simulink model "delay_test"  (R2019a)
settings: Solver=VariableStepAuto  StartTime=0.0  StopTime=512  RelTol=1e-3
libraries: xbsIndex_r4 x3559
(part 1 of 23)
settings Model: Creator=jackh  LastModifiedBy=jackh

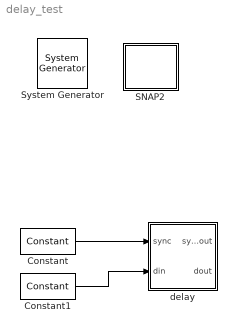
== system delay_test ==
  " System Generator" : xbsIndex_r4/ System Generator  Tag=genX  xilinxfamily=kintexu  part=xcku115  speed=-2-e  package=flvf1924  synthesis_tool=XST  clock_wrapper=Clock Enables  directory=/home/jackh/src/caltech-lwa/snap2_f_200msps_64i_4096c/sysgen  proj_type=Vivado  Synth_file=Vivado Synthesis Defaults  Impl_file=Vivado Implementation Defaults  testbench=off  simulink_period=1  sysclk_period=5  dcm_input_clock_period=10  incr_netlist=off  trim_vbits=Everywhere in SubSystem  dbl_ovrd=According to Block Masks  core_generation=According to Block Masks  run_coregen=off  deprecated_control=off  eval_field=0  block_type=sysgen
  Constant : xbsIndex_r4/Constant  const=0  gui_display_data_type=Boolean  arith_type=Boolean  n_bits=16  bin_pt=14  preci_type=Single  exp_width=8  frac_width=24  explicit_period=on  period=1  equ=P=C  opselect=C  inp2=PCIN>>17  opr=+  inp1=P  carry=CIN  dbl_ovrd=off  block_type=constant
  Constant1 : xbsIndex_r4/Constant  const=0  gui_display_data_type=Fixed-point  arith_type=Unsigned  n_bits=10*64  bin_pt=14  preci_type=Single  exp_width=8  frac_width=24  explicit_period=on  period=1  equ=P=C  opselect=C  inp2=PCIN>>17  opr=+  inp1=P  carry=CIN  dbl_ovrd=off  block_type=constant
  SNAP2 : Subsystem  Tag=xps:xsg  mask(xsg core config){hw_sys=SNAP2_v2:xcku115, clk_src=adc1_clk, clk_rate=200, use_microblaze=on, sample_period=1, synthesis_tool=XST}
      mask prompts: hw_sys "Hardware Platform"; clk_src "User IP Clock source"; clk_rate "User IP Clock Rate (MHz)"; use_microblaze "Use Microblaze controller?"; sample_period "Sample Period"; synthesis_tool "Synthesis Tool:"
      mask help:
      | The XSG Core Config block is used to configure the System Generator design
      | for the casper_xps toolflow. Settings here are used to configure the
      | Xilinx System Generator block parameters automatically, and control toolflow
      | script  execution. It needs to be at the top level of all designs being compiled
      | with the casper_xps toolflow.
      mask init:
      | xps_xsg_snap2_conf_mask;
      mask Help: eval('xlWeb([getenv(''MLIB_ROOT''), ''\doc\html\sys_xsg_core_config\sys_xsg_core_config.html''])')
      mask TypeOptions hw_sys: SNAP2_v1:xcku115 | SNAP2_v2:xcku115
      mask TypeOptions clk_src: sys_clk | clk_250MHz | adc0_clk | adc1_clk
      mask TypeOptions synthesis_tool: Leonardo Spectrum | Synplify | Synplify Pro | XST
      mask Display: fprintf(['SNAP2']);
  delay : Subsystem  mask{max_delay_bits=13}
      mask prompts: max_delay_bits "Manimum delay (2^?) samples"
  wires:
  Constant/1 -> delay/1(sync)
  Constant1/1 -> delay/2(din)

== system delay_test/SNAP2 ==

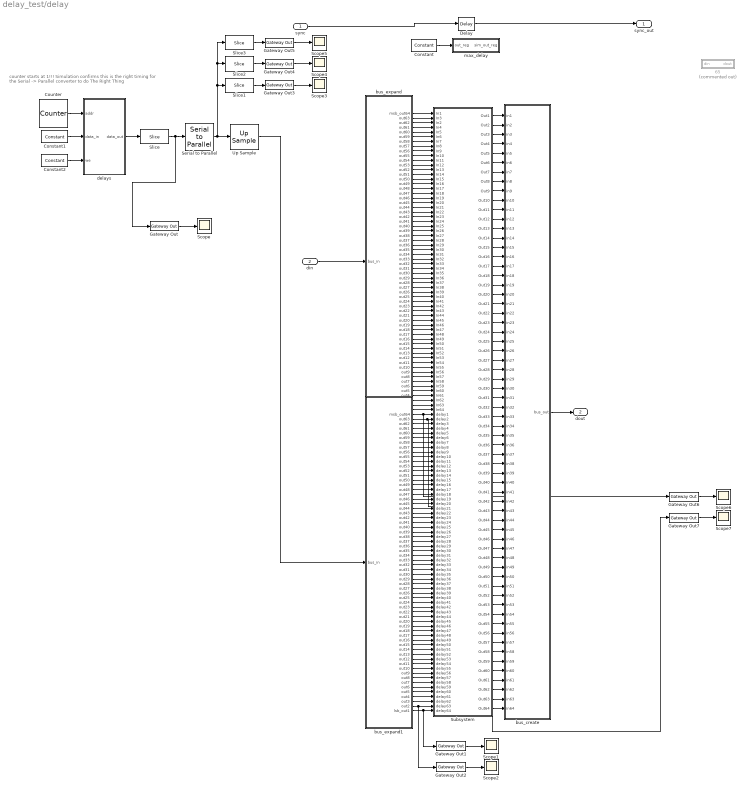
== system delay_test/delay ==
  note: counter starts at 1!!!
      | Simulation confirms this is the right
      | timing for the Serial -> Parallel converter to do The Right Thing
  sync : Inport
  din : Inport  Port=2
  65 : Subsystem  Commented=on
  Constant : xbsIndex_r4/Constant  const=2^max_delay_bits  gui_display_data_type=Fixed-point  arith_type=Unsigned  n_bits=32  bin_pt=0  preci_type=Single  exp_width=8  frac_width=24  explicit_period=on  period=1  equ=P=C  opselect=C  inp2=PCIN>>17  opr=+  inp1=P  carry=CIN  dbl_ovrd=off  block_type=constant
  Constant1 : xbsIndex_r4/Constant  const=0  gui_display_data_type=Fixed-point  arith_type=Unsigned  n_bits=32  bin_pt=0  preci_type=Single  exp_width=8  frac_width=24  explicit_period=on  period=1  equ=P=C  opselect=C  inp2=PCIN>>17  opr=+  inp1=P  carry=CIN  dbl_ovrd=off  block_type=constant
  Constant2 : xbsIndex_r4/Constant  const=0  gui_display_data_type=Boolean  arith_type=Boolean  n_bits=32  bin_pt=0  preci_type=Single  exp_width=8  frac_width=24  explicit_period=on  period=1  equ=P=C  opselect=C  inp2=PCIN>>17  opr=+  inp1=P  carry=CIN  dbl_ovrd=off  block_type=constant
  Counter : xbsIndex_r4/Counter  cnt_type=Free Running  cnt_to=Inf  operation=Up  start_count=1  cnt_by_val=1  arith_type=Unsigned  n_bits=6  bin_pt=0  load_pin=off  rst=off  en=off  explicit_period=on  period=1  use_behavioral_HDL=off  implementation=Fabric  dbl_ovrd=off  block_type=counter
  Delay : xbsIndex_r4/Delay  rst=off  infoeditControl=Selection of Reset will increase slice count due to use of real FFs and instead of SRLs  en=off  latency=7  reg_retiming=on  dbl_ovrd=off  block_type=delay
  Gateway Out{,1..7} (8 alike) : xbsIndex_r4/Gateway Out  inherit_from_input=off  hdl_port=off  rows=1  columns=1  UseAsDAC=off  DACChannel='1'  interface=None  automatic_assignment=on  address_offset=hex2dec('00')  intf_name=''  intf_description=''  timing_constraint=None  locs_specified=off  LOCs={}  io_standard={}  block_type=gatewayout
  Scope{,1..7} (8 alike) : Scope
  Serial to Parallel : xbsIndex_r4/Serial to Parallel  input_order=Most Significant Word First  arith_type=Unsigned  output_bits=13*64  bin_pt=0  rst=off  en=off  latency=1  dbl_ovrd=off  block_type=s2p
      settings: infoedit=Groups of samples presented serially at the input become single samples presented at the output.
  Slice : xbsIndex_r4/Slice  nbits=13  boolean_output=off  mode=Lower Bit Location + Width  bit1=0  base1=MSB of Input  bit0=0  base0=LSB of Input  dbl_ovrd=off  block_type=slice
  Slice1 : xbsIndex_r4/Slice  nbits=13  boolean_output=off  mode=Lower Bit Location + Width  bit1=0  base1=MSB of Input  bit0=0  base0=LSB of Input  dbl_ovrd=off  block_type=slice
  Slice2 : xbsIndex_r4/Slice  nbits=13  boolean_output=off  mode=Lower Bit Location + Width  bit1=0  base1=MSB of Input  bit0=13  base0=LSB of Input  dbl_ovrd=off  block_type=slice
  Slice3 : xbsIndex_r4/Slice  nbits=13  boolean_output=off  mode=Lower Bit Location + Width  bit1=0  base1=MSB of Input  bit0=13*2  base0=LSB of Input  dbl_ovrd=off  block_type=slice
  Subsystem : Subsystem
  Up Sample : xbsIndex_r4/Up Sample  sample_ratio=64  copy_samples=on  en=off  latency=1  dbl_ovrd=off  block_type=usamp
  bus_create : Subsystem  AncestorBlock=casper_library_flow_control/bus_create  mask(bus_create){inputNum=64}
      mask prompts: inputNum "Number of inputs:"
      mask init:
      | bus_create_init(gcb,...
      |     'inputNum', inputNum);
  bus_expand : Subsystem  AncestorBlock=casper_library_flow_control/bus_expand  mask(bus_expand){mode=divisions of equal size, outputNum=8*8, outputWidth=10, outputBinaryPt=0, outputArithmeticType=0, show_format=off, outputToWorkspace=off, variablePrefix=out, outputToModelAsWell=on}
      mask prompts: outputNum "Number of outputs:"; outputWidth "Output width:"; outputBinaryPt "Output binary point position:"; outputArithmeticType "Output arithmetic type (ufix=0, fix=1, bool=2):"; show_format "Print format string?"; outputToWorkspace "Output to workspace?"; variablePrefix "Variable name prefix:"; outputToModelAsWell "Output to model as well?"
      mask help:
      | Expands a 'bus' made using a bus_create or Xilinx
      | concat block.
      | The input will be divided into the specified number
      | of outputs with the specified arithmetic types.
      | Divisions are made from most significant bit.
      mask init:
      | bus_expand_init(gcb,...
      |     'mode', mode, ...
      |     'outputNum', outputNum, ...
      |     'outputWidth', outputWidth, ...
      |     'outputBinaryPt', outputBinaryPt, ...
      |     'outputArithmeticType', outputArithmeticType, ...
      |     'show_format', show_format, ...
      |     'outputToWorkspace', outputToWorkspace, ...
      |     'variablePrefix', variablePrefix, ...
      |     'outputToModelAsWell', outputToModelAsWell);
      settings: AttributesFormatString=64 outputs
      mask TypeOptions mode: divisions of equal size | divisions of arbitrary size
      mask Callback mode: bus_expand_callback();
      mask Callback outputWidth: bus_expand_callback();
      mask Callback outputToWorkspace: bus_expand_callback();
  bus_expand1 : Subsystem  AncestorBlock=casper_library_flow_control/bus_expand  mask(bus_expand){mode=divisions of equal size, outputNum=8*8, outputWidth=13, outputBinaryPt=0, outputArithmeticType=0, show_format=off, outputToWorkspace=off, variablePrefix=out, outputToModelAsWell=on}
      mask prompts: outputNum "Number of outputs:"; outputWidth "Output width:"; outputBinaryPt "Output binary point position:"; outputArithmeticType "Output arithmetic type (ufix=0, fix=1, bool=2):"; show_format "Print format string?"; outputToWorkspace "Output to workspace?"; variablePrefix "Variable name prefix:"; outputToModelAsWell "Output to model as well?"
      mask help:
      | Expands a 'bus' made using a bus_create or Xilinx
      | concat block.
      | The input will be divided into the specified number
      | of outputs with the specified arithmetic types.
      | Divisions are made from most significant bit.
      mask init: same as delay_test/delay/bus_expand
      settings: AttributesFormatString=64 outputs
      mask TypeOptions mode: divisions of equal size | divisions of arbitrary size
      mask Callback mode: bus_expand_callback();
      mask Callback outputWidth: bus_expand_callback();
      mask Callback outputToWorkspace: bus_expand_callback();
  delays : Subsystem  Tag=xps:bram  AncestorBlock=xps_library/Memory/shared_bram  mask{sample_rate=1, init_vals=[0:2^6-1], data_bin_pt=0, optimization=Minimum_Area, reg_core_output=off, reg_prim_output=off, data_width=32, addr_width=6, arith_type=Unsigned, desc_str="", type_desc=""}
      mask prompts: sample_rate "Sample rate"; init_vals "Initial values (simulation only)"; data_bin_pt "Data Binary Point"; reg_core_output "Register Core Output"; reg_prim_output "Register Primitive Output"; data_width "Data Width"; addr_width "Address width"; arith_type "Output Data Type"; desc_str "Description"; type_desc "Word Type Description"
      mask init:
      | shared_bram_mask;
      mask TypeOptions optimization: Minimum_Area | Low_Power
      mask TypeOptions data_width: 8 | 16 | 32 | 64 | 128
      mask TypeOptions arith_type: Unsigned | Signed  (2's comp)
      mask DialogControl Container4 Prompt: Configuration
      mask DialogControl Container10 Prompt: Documentation
  max_delay : Subsystem  Tag=xps:sw_reg  AncestorBlock=xps_library/Memory/software_register  mask(swreg){io_dir=To Processor, io_delay=0, init_val=0, sample_period=1, names=reg, bitwidths=32, bin_pts=0, arith_types=0, sim_port=on, show_format=off, desc_str=|}
      mask desc_str=|
      | Interpretted as a unint32 value, contains the maximum
      | allowed delay, in ADC samples, which may be applied
      | to a data stream.
      mask prompts: io_dir "I/O direction"; io_delay "I/O delay"; init_val "Initial Value"; sample_period "Sample period"; names "Bitfield names [msb...lsb]"; bitwidths "Bitfield widths"; bin_pts "Bitfield binary pts"; arith_types "Bitfield types, ufix=0, fix=1, bool=2"; sim_port "Provide sim input/output?"; show_format "Print format string?"; desc_str "Description"
      mask help: A 32-bit software-accessible register. Can be divided into bitfields of varying widths and types using the fields in the block mask.
      mask init:
      | swreg_init(gcb)
      settings: AttributesFormatString=1output
      mask TypeOptions io_dir: To Processor | From Processor
      mask Callback io_dir:
      | mask_enables = get_param(gcb, 'MaskEnables');
      | mask_names = get_param(gcb, 'MaskNames');
      | if strcmp(get_param(gcb, 'io_dir'), 'To Processor'),
      |     mask_enables{ismember(mask_names, 'sample_period')} = 'off';
      | else
      |     mask_enables{ismember(mask_names, 'sample_period')} = 'on';
      | end
      | set_param(gcb, 'MaskEnables', mask_enables);
      mask DialogControl ParameterTabVar0 Prompt: Setup
  sync_out : Outport
  dout : Outport  Port=2
  wires:
  sync/1 -> Delay/1
  din/1 -> bus_expand/1(bus_in)
  bus_create/1(bus_out) -> dout/1
  Constant/1 -> max_delay/1(out_reg)
  Delay/1 -> sync_out/1
  Counter/1 -> delays/1(addr)
  Constant1/1 -> delays/2(data_in)
  Constant2/1 -> delays/3(we)
  delays/1(data_out) -> Slice/1
  Serial to Parallel/1 -> Up Sample/1, Slice3/1, Slice2/1, Slice1/1
  Slice/1 -> Gateway Out/1, Serial to Parallel/1
  Up Sample/1 -> bus_expand1/1(bus_in)
  Subsystem/1(Out1) -> bus_create/1(in1)
  Subsystem/2(Out2) -> bus_create/2(in2)
  Subsystem/3(Out3) -> bus_create/3(in3)
  Subsystem/4(Out4) -> bus_create/4(in4)
  Subsystem/5(Out5) -> bus_create/5(in5)
  Subsystem/6(Out6) -> bus_create/6(in6)
  Subsystem/7(Out7) -> bus_create/7(in7)
  Subsystem/8(Out8) -> bus_create/8(in8)
  Subsystem/9(Out9) -> bus_create/9(in9)
  Subsystem/10(Out10) -> bus_create/10(in10)
  Subsystem/11(Out11) -> bus_create/11(in11)
  Subsystem/12(Out12) -> bus_create/12(in12)
  Subsystem/13(Out13) -> bus_create/13(in13)
  Subsystem/14(Out14) -> bus_create/14(in14)
  Subsystem/15(Out15) -> bus_create/15(in15)
  Subsystem/16(Out16) -> bus_create/16(in16)
  Subsystem/17(Out17) -> bus_create/17(in17)
  Subsystem/18(Out18) -> bus_create/18(in18)
  Subsystem/19(Out19) -> bus_create/19(in19)
  Subsystem/20(Out20) -> bus_create/20(in20)
  Subsystem/21(Out21) -> bus_create/21(in21)
  Subsystem/22(Out22) -> bus_create/22(in22)
  Subsystem/23(Out23) -> bus_create/23(in23)
  Subsystem/24(Out24) -> bus_create/24(in24)
  Subsystem/25(Out25) -> bus_create/25(in25)
  Subsystem/26(Out26) -> bus_create/26(in26)
  Subsystem/27(Out27) -> bus_create/27(in27)
  Subsystem/28(Out28) -> bus_create/28(in28)
  Subsystem/29(Out29) -> bus_create/29(in29)
  Subsystem/30(Out30) -> bus_create/30(in30)
  Subsystem/31(Out31) -> bus_create/31(in31)
  Subsystem/32(Out32) -> bus_create/32(in32)
  Subsystem/33(Out33) -> bus_create/33(in33)
  Subsystem/34(Out34) -> bus_create/34(in34)
  Subsystem/35(Out35) -> bus_create/35(in35)
  Subsystem/36(Out36) -> bus_create/36(in36)
  Subsystem/37(Out37) -> bus_create/37(in37)
  Subsystem/38(Out38) -> bus_create/38(in38)
  Subsystem/39(Out39) -> bus_create/39(in39)
  Subsystem/40(Out40) -> bus_create/40(in40)
  Subsystem/41(Out41) -> bus_create/41(in41)
  Subsystem/42(Out42) -> bus_create/42(in42)
  Subsystem/43(Out43) -> bus_create/43(in43)
  Subsystem/44(Out44) -> bus_create/44(in44)
  Subsystem/45(Out45) -> bus_create/45(in45)
  Subsystem/46(Out46) -> bus_create/46(in46)
  Subsystem/47(Out47) -> bus_create/47(in47)
  Subsystem/48(Out48) -> bus_create/48(in48)
  Subsystem/49(Out49) -> bus_create/49(in49)
  Subsystem/50(Out50) -> bus_create/50(in50)
  Subsystem/51(Out51) -> bus_create/51(in51)
  Subsystem/52(Out52) -> bus_create/52(in52)
  Subsystem/53(Out53) -> bus_create/53(in53)
  Subsystem/54(Out54) -> bus_create/54(in54)
  Subsystem/55(Out55) -> bus_create/55(in55)
  Subsystem/56(Out56) -> bus_create/56(in56)
  Subsystem/57(Out57) -> bus_create/57(in57)
  Subsystem/58(Out58) -> bus_create/58(in58)
  Subsystem/59(Out59) -> bus_create/59(in59)
  Subsystem/60(Out60) -> bus_create/60(in60)
  Subsystem/61(Out61) -> bus_create/61(in61)
  Subsystem/62(Out62) -> bus_create/62(in62)
  Subsystem/63(Out63) -> bus_create/63(in63)
  Subsystem/64(Out64) -> bus_create/64(in64)
  bus_expand/1(msb_out64) -> Subsystem/1(In1)
  bus_expand/2(out63) -> Subsystem/2(In3)
  bus_expand/3(out62) -> Subsystem/3(In2)
  bus_expand/4(out61) -> Subsystem/4(In4)
  bus_expand/5(out60) -> Subsystem/5(In5)
  bus_expand/6(out59) -> Subsystem/6(In6)
  bus_expand/7(out58) -> Subsystem/7(In7)
  bus_expand/8(out57) -> Subsystem/8(In8)
  bus_expand/9(out56) -> Subsystem/9(In9)
  bus_expand/10(out55) -> Subsystem/10(In10)
  bus_expand/11(out54) -> Subsystem/11(In11)
  bus_expand/12(out53) -> Subsystem/12(In12)
  bus_expand/13(out52) -> Subsystem/13(In13)
  bus_expand/14(out51) -> Subsystem/14(In14)
  bus_expand/15(out50) -> Subsystem/15(In15)
  bus_expand/16(out49) -> Subsystem/16(In16)
  bus_expand/17(out48) -> Subsystem/17(In17)
  bus_expand/18(out47) -> Subsystem/18(In18)
  bus_expand/19(out46) -> Subsystem/19(In19)
  bus_expand/20(out45) -> Subsystem/20(In20)
  bus_expand/21(out44) -> Subsystem/21(In21)
  bus_expand/22(out43) -> Subsystem/22(In22)
  bus_expand/23(out42) -> Subsystem/23(In23)
  bus_expand/24(out41) -> Subsystem/24(In24)
  bus_expand/25(out40) -> Subsystem/25(In25)
  bus_expand/26(out39) -> Subsystem/26(In26)
  bus_expand/27(out38) -> Subsystem/27(In27)
  bus_expand/28(out37) -> Subsystem/28(In28)
  bus_expand/29(out36) -> Subsystem/29(In29)
  bus_expand/30(out35) -> Subsystem/30(In30)
  bus_expand/31(out34) -> Subsystem/31(In31)
  bus_expand/32(out33) -> Subsystem/32(In32)
  bus_expand/33(out32) -> Subsystem/33(In33)
  bus_expand/34(out31) -> Subsystem/34(In34)
  bus_expand/35(out30) -> Subsystem/35(In35)
  bus_expand/36(out29) -> Subsystem/36(In36)
  bus_expand/37(out28) -> Subsystem/37(In37)
  bus_expand/38(out27) -> Subsystem/38(In38)
  bus_expand/39(out26) -> Subsystem/39(In39)
  bus_expand/40(out25) -> Subsystem/40(In40)
  bus_expand/41(out24) -> Subsystem/41(In41)
  bus_expand/42(out23) -> Subsystem/42(In42)
  bus_expand/43(out22) -> Subsystem/43(In43)
  bus_expand/44(out21) -> Subsystem/44(In44)
  bus_expand/45(out20) -> Subsystem/45(In45)
  bus_expand/46(out19) -> Subsystem/46(In46)
  bus_expand/47(out18) -> Subsystem/47(In47)
  bus_expand/48(out17) -> Subsystem/48(In48)
  bus_expand/49(out16) -> Subsystem/49(In49)
  bus_expand/50(out15) -> Subsystem/50(In50)
  bus_expand/51(out14) -> Subsystem/51(In51)
  bus_expand/52(out13) -> Subsystem/52(In52)
  bus_expand/53(out12) -> Subsystem/53(In53)
  bus_expand/54(out11) -> Subsystem/54(In54)
  bus_expand/55(out10) -> Subsystem/55(In55)
  bus_expand/56(out9) -> Subsystem/56(In56)
  bus_expand/57(out8) -> Subsystem/57(In57)
  bus_expand/58(out7) -> Subsystem/58(In58)
  bus_expand/59(out6) -> Subsystem/59(In59)
  bus_expand/60(out5) -> Subsystem/60(In60)
  bus_expand/61(out4) -> Subsystem/61(In61)
  bus_expand/62(out3) -> Subsystem/62(In62)
  bus_expand/63(out2) -> Subsystem/63(In63)
  bus_expand/64(lsb_out1) -> Subsystem/64(In64)
  bus_expand1/1(msb_out64) -> Gateway Out6/1, Subsystem/65(delay1)
  bus_expand1/2(out63) -> Gateway Out7/1, Subsystem/66(delay2)
  bus_expand1/3(out62) -> Subsystem/67(delay3)
  bus_expand1/4(out61) -> Subsystem/68(delay4)
  bus_expand1/5(out60) -> Subsystem/69(delay5)
  bus_expand1/6(out59) -> Subsystem/70(delay6)
  bus_expand1/7(out58) -> Subsystem/71(delay7)
  bus_expand1/8(out57) -> Subsystem/72(delay8)
  bus_expand1/9(out56) -> Subsystem/73(delay9)
  bus_expand1/10(out55) -> Subsystem/74(delay10)
  bus_expand1/11(out54) -> Subsystem/75(delay11)
  bus_expand1/12(out53) -> Subsystem/76(delay12)
  bus_expand1/13(out52) -> Subsystem/77(delay13)
  bus_expand1/14(out51) -> Subsystem/78(delay14)
  bus_expand1/15(out50) -> Subsystem/79(delay15)
  bus_expand1/16(out49) -> Subsystem/80(delay16)
  bus_expand1/17(out48) -> Subsystem/81(delay17)
  bus_expand1/18(out47) -> Subsystem/82(delay18)
  bus_expand1/19(out46) -> Subsystem/83(delay19)
  bus_expand1/20(out45) -> Subsystem/84(delay20)
  bus_expand1/21(out44) -> Subsystem/85(delay21)
  bus_expand1/22(out43) -> Subsystem/86(delay22)
  bus_expand1/23(out42) -> Subsystem/87(delay23)
  bus_expand1/24(out41) -> Subsystem/88(delay24)
  bus_expand1/25(out40) -> Subsystem/89(delay25)
  bus_expand1/26(out39) -> Subsystem/90(delay26)
  bus_expand1/27(out38) -> Subsystem/91(delay27)
  bus_expand1/28(out37) -> Subsystem/92(delay28)
  bus_expand1/29(out36) -> Subsystem/93(delay29)
  bus_expand1/30(out35) -> Subsystem/94(delay30)
  bus_expand1/31(out34) -> Subsystem/95(delay31)
  bus_expand1/32(out33) -> Subsystem/96(delay32)
  bus_expand1/33(out32) -> Subsystem/97(delay33)
  bus_expand1/34(out31) -> Subsystem/98(delay34)
  bus_expand1/35(out30) -> Subsystem/99(delay35)
  bus_expand1/36(out29) -> Subsystem/100(delay36)
  bus_expand1/37(out28) -> Subsystem/101(delay37)
  bus_expand1/38(out27) -> Subsystem/102(delay38)
  bus_expand1/39(out26) -> Subsystem/103(delay39)
  bus_expand1/40(out25) -> Subsystem/104(delay40)
  bus_expand1/41(out24) -> Subsystem/105(delay41)
  bus_expand1/42(out23) -> Subsystem/106(delay42)
  bus_expand1/43(out22) -> Subsystem/107(delay43)
  bus_expand1/44(out21) -> Subsystem/108(delay44)
  bus_expand1/45(out20) -> Subsystem/109(delay45)
  bus_expand1/46(out19) -> Subsystem/110(delay46)
  bus_expand1/47(out18) -> Subsystem/111(delay47)
  bus_expand1/48(out17) -> Subsystem/112(delay48)
  bus_expand1/49(out16) -> Subsystem/113(delay49)
  bus_expand1/50(out15) -> Subsystem/114(delay50)
  bus_expand1/51(out14) -> Subsystem/115(delay51)
  bus_expand1/52(out13) -> Subsystem/116(delay52)
  bus_expand1/53(out12) -> Subsystem/117(delay53)
  bus_expand1/54(out11) -> Subsystem/118(delay54)
  bus_expand1/55(out10) -> Subsystem/119(delay55)
  bus_expand1/56(out9) -> Subsystem/120(delay56)
  bus_expand1/57(out8) -> Subsystem/121(delay57)
  bus_expand1/58(out7) -> Subsystem/122(delay58)
  bus_expand1/59(out6) -> Subsystem/123(delay59)
  bus_expand1/60(out5) -> Subsystem/124(delay60)
  bus_expand1/61(out4) -> Subsystem/125(delay61)
  bus_expand1/62(out3) -> Subsystem/126(delay62)
  bus_expand1/63(out2) -> Gateway Out2/1, Subsystem/127(delay63)
  bus_expand1/64(lsb_out1) -> Gateway Out1/1, Subsystem/128(delay64)
  Gateway Out/1 -> Scope/1
  Gateway Out1/1 -> Scope1/1
  Gateway Out2/1 -> Scope2/1
  Gateway Out3/1 -> Scope3/1
  Slice1/1 -> Gateway Out3/1
  Slice2/1 -> Gateway Out4/1
  Gateway Out4/1 -> Scope4/1
  Gateway Out5/1 -> Scope5/1
  Slice3/1 -> Gateway Out5/1
  Gateway Out7/1 -> Scope7/1
  Gateway Out6/1 -> Scope6/1

== system delay_test/delay/65 ==
  din : Inport
  Slice : xbsIndex_r4/Slice  nbits=10  boolean_output=off  mode=Lower Bit Location + Width  bit1=0  base1=MSB of Input  bit0=0  base0=LSB of Input  dbl_ovrd=off  block_type=slice
  Slice1 : xbsIndex_r4/Slice  nbits=3  boolean_output=off  mode=Lower Bit Location + Width  bit1=0  base1=MSB of Input  bit0=10  base0=LSB of Input  dbl_ovrd=off  block_type=slice
  Subsystem1 : Subsystem
  delay : Subsystem  Tag=xps:sw_reg  AncestorBlock=xps_library/Memory/software_register  mask(swreg){io_dir=From Processor, io_delay=0, init_val=0, sample_period=1, names=reg, bitwidths=13, bin_pts=0, arith_types=0, sim_port=on, show_format=off, desc_str=|}
      mask desc_str=|
      | The delay applied to stream ``n``, where the register
      | name has suffix ``<n>_delay``.
      | Any value entered in this 32-bit register will be
      | interpretted modulo the maximum supported delay.
      mask prompts: io_dir "I/O direction"; io_delay "I/O delay"; init_val "Initial Value"; sample_period "Sample period"; names "Bitfield names [msb...lsb]"; bitwidths "Bitfield widths"; bin_pts "Bitfield binary pts"; arith_types "Bitfield types, ufix=0, fix=1, bool=2"; sim_port "Provide sim input/output?"; show_format "Print format string?"; desc_str "Description"
      mask help: A 32-bit software-accessible register. Can be divided into bitfields of varying widths and types using the fields in the block mask.
      mask init:
      | swreg_init(gcb)
      settings: AttributesFormatString=1input
      mask TypeOptions io_dir: To Processor | From Processor
      mask Callback io_dir:
      | mask_enables = get_param(gcb, 'MaskEnables');
      | mask_names = get_param(gcb, 'MaskNames');
      | if strcmp(get_param(gcb, 'io_dir'), 'To Processor'),
      |     mask_enables{ismember(mask_names, 'sample_period')} = 'off';
      | else
      |     mask_enables{ismember(mask_names, 'sample_period')} = 'on';
      | end
      | set_param(gcb, 'MaskEnables', mask_enables);
      mask DialogControl ParameterTabVar0 Prompt: Setup
  delay_bram_prog_dp : Subsystem  AncestorBlock=casper_library_delays/delay_bram_prog_dp  mask(delay_bram_prog_dp){ram_bits=max_delay_bits-3, bram_latency=2, async=off}
      mask prompts: ram_bits "Max delay (2^?)"; bram_latency "BRAM latency"; async "asynchronous operation"
      mask init:
      | delay_bram_prog_dp_init(gcb, ...
      |     'ram_bits', ram_bits, ...
      |     'bram_latency', bram_latency, ...
      |     'async', async);
  dout : Outport
  wires:
  Subsystem1/1(dout) -> dout/1
  delay_bram_prog_dp/1(dout) -> Subsystem1/1(din)
  Slice1/1 -> Subsystem1/2(delay)
  Slice/1 -> delay_bram_prog_dp/2(delay)
  delay/1(in_reg) -> Slice/1, Slice1/1
  din/1 -> delay_bram_prog_dp/1(din)

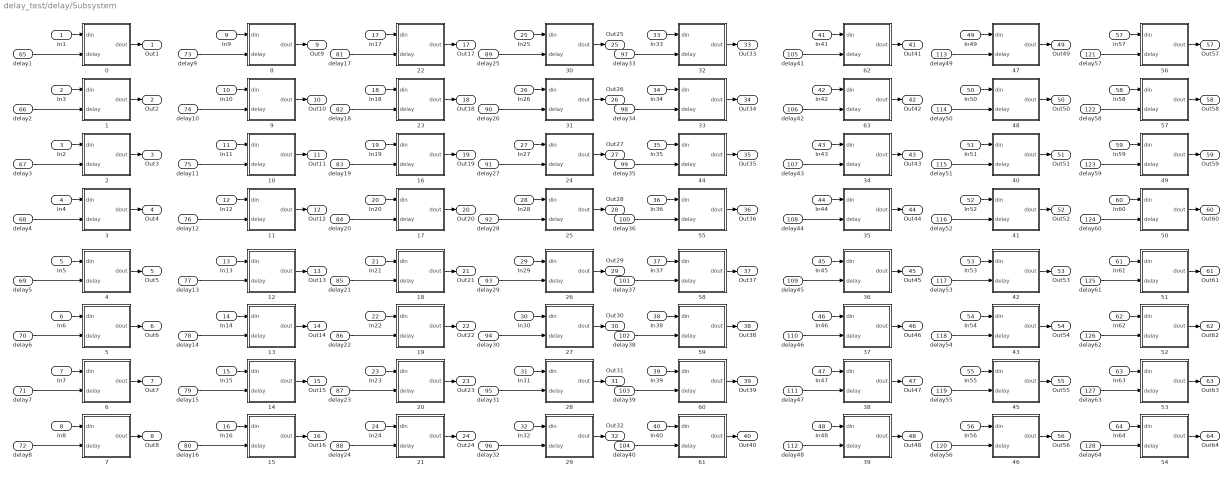
== system delay_test/delay/Subsystem ==
  In1 : Inport
  In3 : Inport  Port=2
  In2 : Inport  Port=3
  In4 : Inport  Port=4
  In5 : Inport  Port=5
  In6 : Inport  Port=6
  In7 : Inport  Port=7
  In8 : Inport  Port=8
  In9 : Inport  Port=9
  In10 : Inport  Port=10
  In11 : Inport  Port=11
  In12 : Inport  Port=12
  In13 : Inport  Port=13
  In14 : Inport  Port=14
  In15 : Inport  Port=15
  In16 : Inport  Port=16
  In17 : Inport  Port=17
  In18 : Inport  Port=18
  In19 : Inport  Port=19
  In20 : Inport  Port=20
  In21 : Inport  Port=21
  In22 : Inport  Port=22
  In23 : Inport  Port=23
  In24 : Inport  Port=24
  In25 : Inport  Port=25
  In26 : Inport  Port=26
  In27 : Inport  Port=27
  In28 : Inport  Port=28
  In29 : Inport  Port=29
  In30 : Inport  Port=30
  In31 : Inport  Port=31
  In32 : Inport  Port=32
  In33 : Inport  Port=33
  In34 : Inport  Port=34
  In35 : Inport  Port=35
  In36 : Inport  Port=36
  In37 : Inport  Port=37
  In38 : Inport  Port=38
  In39 : Inport  Port=39
  In40 : Inport  Port=40
  In41 : Inport  Port=41
  In42 : Inport  Port=42
  In43 : Inport  Port=43
  In44 : Inport  Port=44
  In45 : Inport  Port=45
  In46 : Inport  Port=46
  In47 : Inport  Port=47
  In48 : Inport  Port=48
  In49 : Inport  Port=49
  In50 : Inport  Port=50
  In51 : Inport  Port=51
  In52 : Inport  Port=52
  In53 : Inport  Port=53
  In54 : Inport  Port=54
  In55 : Inport  Port=55
  In56 : Inport  Port=56
  In57 : Inport  Port=57
  In58 : Inport  Port=58
  In59 : Inport  Port=59
  In60 : Inport  Port=60
  In61 : Inport  Port=61
  In62 : Inport  Port=62
  In63 : Inport  Port=63
  In64 : Inport  Port=64
  delay1 : Inport  Port=65
  delay2 : Inport  Port=66
  delay3 : Inport  Port=67
  delay4 : Inport  Port=68
  delay5 : Inport  Port=69
  delay6 : Inport  Port=70
  delay7 : Inport  Port=71
  delay8 : Inport  Port=72
  delay9 : Inport  Port=73
  delay10 : Inport  Port=74
  delay11 : Inport  Port=75
  delay12 : Inport  Port=76
  delay13 : Inport  Port=77
  delay14 : Inport  Port=78
  delay15 : Inport  Port=79
  delay16 : Inport  Port=80
  delay17 : Inport  Port=81
  delay18 : Inport  Port=82
  delay19 : Inport  Port=83
  delay20 : Inport  Port=84
  delay21 : Inport  Port=85
  delay22 : Inport  Port=86
  delay23 : Inport  Port=87
  delay24 : Inport  Port=88
  delay25 : Inport  Port=89
  delay26 : Inport  Port=90
  delay27 : Inport  Port=91
  delay28 : Inport  Port=92
  delay29 : Inport  Port=93
  delay30 : Inport  Port=94
  delay31 : Inport  Port=95
  delay32 : Inport  Port=96
  delay33 : Inport  Port=97
  delay34 : Inport  Port=98
  delay35 : Inport  Port=99
  delay36 : Inport  Port=100
  delay37 : Inport  Port=101
  delay38 : Inport  Port=102
  delay39 : Inport  Port=103
  delay40 : Inport  Port=104
  delay41 : Inport  Port=105
  delay42 : Inport  Port=106
  delay43 : Inport  Port=107
  delay44 : Inport  Port=108
  delay45 : Inport  Port=109
  delay46 : Inport  Port=110
  delay47 : Inport  Port=111
  delay48 : Inport  Port=112
  delay49 : Inport  Port=113
  delay50 : Inport  Port=114
  delay51 : Inport  Port=115
  delay52 : Inport  Port=116
  delay53 : Inport  Port=117
  delay54 : Inport  Port=118
  delay55 : Inport  Port=119
  delay56 : Inport  Port=120
  delay57 : Inport  Port=121
  delay58 : Inport  Port=122
  delay59 : Inport  Port=123
  delay60 : Inport  Port=124
  delay61 : Inport  Port=125
  delay62 : Inport  Port=126
  delay63 : Inport  Port=127
  delay64 : Inport  Port=128
  0 : Subsystem
  1 : Subsystem
  10 : Subsystem
  11 : Subsystem
  12 : Subsystem
  13 : Subsystem
  14 : Subsystem
  15 : Subsystem
  16 : Subsystem
  17 : Subsystem
  18 : Subsystem
  19 : Subsystem
  2 : Subsystem
  20 : Subsystem
  21 : Subsystem
  22 : Subsystem
  23 : Subsystem
  24 : Subsystem
  25 : Subsystem
  26 : Subsystem
  27 : Subsystem
  28 : Subsystem
  29 : Subsystem
  3 : Subsystem
  30 : Subsystem
  31 : Subsystem
  32 : Subsystem
  33 : Subsystem
  34 : Subsystem
  35 : Subsystem
  36 : Subsystem
  37 : Subsystem
  38 : Subsystem
  39 : Subsystem
  4 : Subsystem
  40 : Subsystem
  41 : Subsystem
  42 : Subsystem
  43 : Subsystem
  44 : Subsystem
  45 : Subsystem
  46 : Subsystem
  47 : Subsystem
  48 : Subsystem
  49 : Subsystem
  5 : Subsystem
  50 : Subsystem
  51 : Subsystem
  52 : Subsystem
  53 : Subsystem
  54 : Subsystem
  55 : Subsystem
  56 : Subsystem
  57 : Subsystem
  58 : Subsystem
  59 : Subsystem
  6 : Subsystem
  60 : Subsystem
  61 : Subsystem
  62 : Subsystem
  63 : Subsystem
  7 : Subsystem
  8 : Subsystem
  9 : Subsystem
  Out1 : Outport
  Out2 : Outport  Port=2
  Out3 : Outport  Port=3
  Out4 : Outport  Port=4
  Out5 : Outport  Port=5
  Out6 : Outport  Port=6
  Out7 : Outport  Port=7
  Out8 : Outport  Port=8
  Out9 : Outport  Port=9
  Out10 : Outport  Port=10
  Out11 : Outport  Port=11
  Out12 : Outport  Port=12
  Out13 : Outport  Port=13
  Out14 : Outport  Port=14
  Out15 : Outport  Port=15
  Out16 : Outport  Port=16
  Out17 : Outport  Port=17
  Out18 : Outport  Port=18
  Out19 : Outport  Port=19
  Out20 : Outport  Port=20
  Out21 : Outport  Port=21
  Out22 : Outport  Port=22
  Out23 : Outport  Port=23
  Out24 : Outport  Port=24
  Out25 : Outport  Port=25
  Out26 : Outport  Port=26
  Out27 : Outport  Port=27
  Out28 : Outport  Port=28
  Out29 : Outport  Port=29
  Out30 : Outport  Port=30
  Out31 : Outport  Port=31
  Out32 : Outport  Port=32
  Out33 : Outport  Port=33
  Out34 : Outport  Port=34
  Out35 : Outport  Port=35
  Out36 : Outport  Port=36
  Out37 : Outport  Port=37
  Out38 : Outport  Port=38
  Out39 : Outport  Port=39
  Out40 : Outport  Port=40
  Out41 : Outport  Port=41
  Out42 : Outport  Port=42
  Out43 : Outport  Port=43
  Out44 : Outport  Port=44
  Out45 : Outport  Port=45
  Out46 : Outport  Port=46
  Out47 : Outport  Port=47
  Out48 : Outport  Port=48
  Out49 : Outport  Port=49
  Out50 : Outport  Port=50
  Out51 : Outport  Port=51
  Out52 : Outport  Port=52
  Out53 : Outport  Port=53
  Out54 : Outport  Port=54
  Out55 : Outport  Port=55
  Out56 : Outport  Port=56
  Out57 : Outport  Port=57
  Out58 : Outport  Port=58
  Out59 : Outport  Port=59
  Out60 : Outport  Port=60
  Out61 : Outport  Port=61
  Out62 : Outport  Port=62
  Out63 : Outport  Port=63
  Out64 : Outport  Port=64
  wires:
  0/1(dout) -> Out1/1
  In1/1 -> 0/1(din)
  In3/1 -> 1/1(din)
  1/1(dout) -> Out2/1
  3/1(dout) -> Out4/1
  In4/1 -> 3/1(din)
  In2/1 -> 2/1(din)
  2/1(dout) -> Out3/1
  6/1(dout) -> Out7/1
  In7/1 -> 6/1(din)
  In8/1 -> 7/1(din)
  7/1(dout) -> Out8/1
  5/1(dout) -> Out6/1
  In6/1 -> 5/1(din)
  In5/1 -> 4/1(din)
  4/1(dout) -> Out5/1
  12/1(dout) -> Out13/1
  In13/1 -> 12/1(din)
  In14/1 -> 13/1(din)
  13/1(dout) -> Out14/1
  15/1(dout) -> Out16/1
  In16/1 -> 15/1(din)
  In15/1 -> 14/1(din)
  14/1(dout) -> Out15/1
  10/1(dout) -> Out11/1
  In11/1 -> 10/1(din)
  In12/1 -> 11/1(din)
  11/1(dout) -> Out12/1
  9/1(dout) -> Out10/1
  In10/1 -> 9/1(din)
  In9/1 -> 8/1(din)
  8/1(dout) -> Out9/1
  22/1(dout) -> Out17/1
  In17/1 -> 22/1(din)
  In18/1 -> 23/1(din)
  23/1(dout) -> Out18/1
  17/1(dout) -> Out20/1
  In20/1 -> 17/1(din)
  In19/1 -> 16/1(din)
  16/1(dout) -> Out19/1
  20/1(dout) -> Out23/1
  In23/1 -> 20/1(din)
  In24/1 -> 21/1(din)
  21/1(dout) -> Out24/1
  19/1(dout) -> Out22/1
  In22/1 -> 19/1(din)
  In21/1 -> 18/1(din)
  18/1(dout) -> Out21/1
  26/1(dout) -> Out29/1
  In29/1 -> 26/1(din)
  In30/1 -> 27/1(din)
  27/1(dout) -> Out30/1
  29/1(dout) -> Out32/1
  In32/1 -> 29/1(din)
  In31/1 -> 28/1(din)
  28/1(dout) -> Out31/1
  24/1(dout) -> Out27/1
  In27/1 -> 24/1(din)
  In28/1 -> 25/1(din)
  25/1(dout) -> Out28/1
  31/1(dout) -> Out26/1
  In26/1 -> 31/1(din)
  In25/1 -> 30/1(din)
  30/1(dout) -> Out25/1
  56/1(dout) -> Out57/1
  In57/1 -> 56/1(din)
  In58/1 -> 57/1(din)
  57/1(dout) -> Out58/1
  50/1(dout) -> Out60/1
  In60/1 -> 50/1(din)
  In59/1 -> 49/1(din)
  49/1(dout) -> Out59/1
  53/1(dout) -> Out63/1
  In63/1 -> 53/1(din)
  In64/1 -> 54/1(din)
  54/1(dout) -> Out64/1
  52/1(dout) -> Out62/1
  In62/1 -> 52/1(din)
  In61/1 -> 51/1(din)
  51/1(dout) -> Out61/1
  42/1(dout) -> Out53/1
  In53/1 -> 42/1(din)
  In54/1 -> 43/1(din)
  43/1(dout) -> Out54/1
  46/1(dout) -> Out56/1
  In56/1 -> 46/1(din)
  In55/1 -> 45/1(din)
  45/1(dout) -> Out55/1
  40/1(dout) -> Out51/1
  In51/1 -> 40/1(din)
  In52/1 -> 41/1(din)
  41/1(dout) -> Out52/1
  48/1(dout) -> Out50/1
  In50/1 -> 48/1(din)
  In49/1 -> 47/1(din)
  47/1(dout) -> Out49/1
  62/1(dout) -> Out41/1
  In41/1 -> 62/1(din)
  In42/1 -> 63/1(din)
  63/1(dout) -> Out42/1
  35/1(dout) -> Out44/1
  In44/1 -> 35/1(din)
  In43/1 -> 34/1(din)
  34/1(dout) -> Out43/1
  38/1(dout) -> Out47/1
  In47/1 -> 38/1(din)
  In48/1 -> 39/1(din)
  39/1(dout) -> Out48/1
  37/1(dout) -> Out46/1
  In46/1 -> 37/1(din)
  In45/1 -> 36/1(din)
  36/1(dout) -> Out45/1
  58/1(dout) -> Out37/1
  In37/1 -> 58/1(din)
  In38/1 -> 59/1(din)
  59/1(dout) -> Out38/1
  61/1(dout) -> Out40/1
  In40/1 -> 61/1(din)
  In39/1 -> 60/1(din)
  60/1(dout) -> Out39/1
  44/1(dout) -> Out35/1
  In35/1 -> 44/1(din)
  In36/1 -> 55/1(din)
  55/1(dout) -> Out36/1
  33/1(dout) -> Out34/1
  In34/1 -> 33/1(din)
  In33/1 -> 32/1(din)
  32/1(dout) -> Out33/1
  delay1/1 -> 0/2(delay)
  delay2/1 -> 1/2(delay)
  delay3/1 -> 2/2(delay)
  delay4/1 -> 3/2(delay)
  delay8/1 -> 7/2(delay)
  delay7/1 -> 6/2(delay)
  delay6/1 -> 5/2(delay)
  delay5/1 -> 4/2(delay)
  delay13/1 -> 12/2(delay)
  delay14/1 -> 13/2(delay)
  delay15/1 -> 14/2(delay)
  delay16/1 -> 15/2(delay)
  delay12/1 -> 11/2(delay)
  delay11/1 -> 10/2(delay)
  delay10/1 -> 9/2(delay)
  delay9/1 -> 8/2(delay)
  delay17/1 -> 22/2(delay)
  delay18/1 -> 23/2(delay)
  delay19/1 -> 16/2(delay)
  delay20/1 -> 17/2(delay)
  delay24/1 -> 21/2(delay)
  delay23/1 -> 20/2(delay)
  delay22/1 -> 19/2(delay)
  delay21/1 -> 18/2(delay)
  delay29/1 -> 26/2(delay)
  delay30/1 -> 27/2(delay)
  delay31/1 -> 28/2(delay)
  delay32/1 -> 29/2(delay)
  delay28/1 -> 25/2(delay)
  delay27/1 -> 24/2(delay)
  delay26/1 -> 31/2(delay)
  delay25/1 -> 30/2(delay)
  delay33/1 -> 32/2(delay)
  delay34/1 -> 33/2(delay)
  delay35/1 -> 44/2(delay)
  delay36/1 -> 55/2(delay)
  delay40/1 -> 61/2(delay)
  delay39/1 -> 60/2(delay)
  delay38/1 -> 59/2(delay)
  delay37/1 -> 58/2(delay)
  delay45/1 -> 36/2(delay)
  delay46/1 -> 37/2(delay)
  delay47/1 -> 38/2(delay)
  delay48/1 -> 39/2(delay)
  delay44/1 -> 35/2(delay)
  delay43/1 -> 34/2(delay)
  delay42/1 -> 63/2(delay)
  delay41/1 -> 62/2(delay)
  delay49/1 -> 47/2(delay)
  delay50/1 -> 48/2(delay)
  delay51/1 -> 40/2(delay)
  delay52/1 -> 41/2(delay)
  delay56/1 -> 46/2(delay)
  delay55/1 -> 45/2(delay)
  delay54/1 -> 43/2(delay)
  delay53/1 -> 42/2(delay)
  delay61/1 -> 51/2(delay)
  delay62/1 -> 52/2(delay)
  delay63/1 -> 53/2(delay)
  delay64/1 -> 54/2(delay)
  delay60/1 -> 50/2(delay)
  delay59/1 -> 49/2(delay)
  delay58/1 -> 57/2(delay)
  delay57/1 -> 56/2(delay)

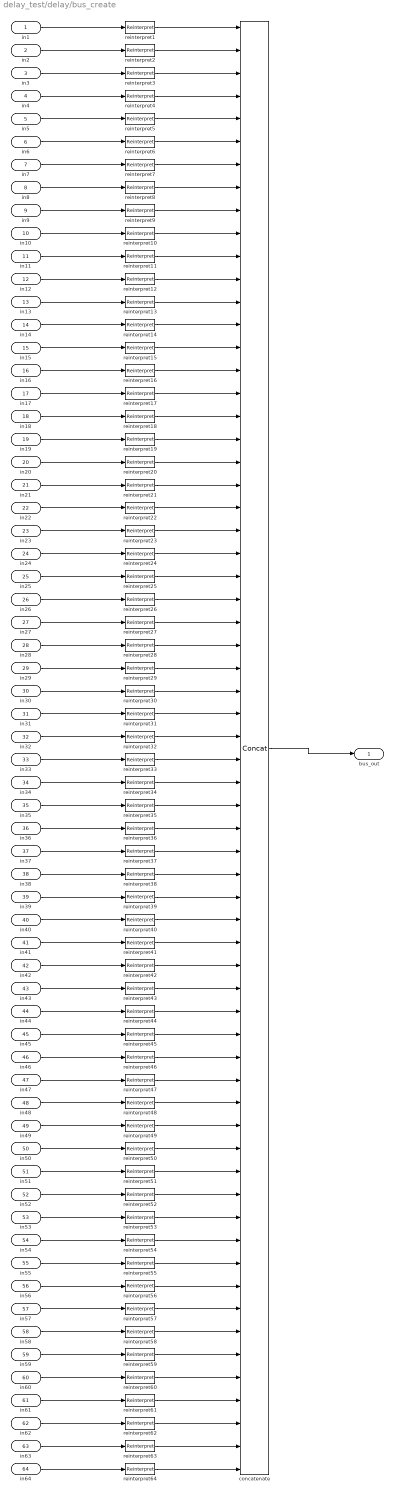
== system delay_test/delay/bus_create ==
  in1 : Inport
  in2 : Inport  Port=2
  in3 : Inport  Port=3
  in4 : Inport  Port=4
  in5 : Inport  Port=5
  in6 : Inport  Port=6
  in7 : Inport  Port=7
  in8 : Inport  Port=8
  in9 : Inport  Port=9
  in10 : Inport  Port=10
  in11 : Inport  Port=11
  in12 : Inport  Port=12
  in13 : Inport  Port=13
  in14 : Inport  Port=14
  in15 : Inport  Port=15
  in16 : Inport  Port=16
  in17 : Inport  Port=17
  in18 : Inport  Port=18
  in19 : Inport  Port=19
  in20 : Inport  Port=20
  in21 : Inport  Port=21
  in22 : Inport  Port=22
  in23 : Inport  Port=23
  in24 : Inport  Port=24
  in25 : Inport  Port=25
  in26 : Inport  Port=26
  in27 : Inport  Port=27
  in28 : Inport  Port=28
  in29 : Inport  Port=29
  in30 : Inport  Port=30
  in31 : Inport  Port=31
  in32 : Inport  Port=32
  in33 : Inport  Port=33
  in34 : Inport  Port=34
  in35 : Inport  Port=35
  in36 : Inport  Port=36
  in37 : Inport  Port=37
  in38 : Inport  Port=38
  in39 : Inport  Port=39
  in40 : Inport  Port=40
  in41 : Inport  Port=41
  in42 : Inport  Port=42
  in43 : Inport  Port=43
  in44 : Inport  Port=44
  in45 : Inport  Port=45
  in46 : Inport  Port=46
  in47 : Inport  Port=47
  in48 : Inport  Port=48
  in49 : Inport  Port=49
  in50 : Inport  Port=50
  in51 : Inport  Port=51
  in52 : Inport  Port=52
  in53 : Inport  Port=53
  in54 : Inport  Port=54
  in55 : Inport  Port=55
  in56 : Inport  Port=56
  in57 : Inport  Port=57
  in58 : Inport  Port=58
  in59 : Inport  Port=59
  in60 : Inport  Port=60
  in61 : Inport  Port=61
  in62 : Inport  Port=62
  in63 : Inport  Port=63
  in64 : Inport  Port=64
  concatenate : xbsIndex_r4/Concat  num_inputs=64  dbl_ovrd=off  block_type=concat
  reinterpret{1..64} (64 alike) : xbsIndex_r4/Reinterpret  force_arith_type=on  arith_type=Unsigned  force_bin_pt=on  bin_pt=0  block_type=reinterpret
      reinterpret1 settings: infoedit="Changes signal type without altering the binary representation.   You can changed the signal between signed and unsigned, and relocate the binary point.<br><br>Hardware notes: In hardware this block costs nothing.<br><br>Example:  Suppose the input is 6 bits wide, signed, with 2 fractional bits, and the output is forced to unsigned with 0 fractional bits.  Then an input of -2.0 (1110.00 in binary 2's complement) becomes an output of 56 (111000 in binary)."
      reinterpret2 settings: infoedit="Changes signal type without altering the binary representation.   You can changed the signal between signed and unsigned, and relocate the binary point.<br><br>Hardware notes: In hardware this block costs nothing.<br><br>Example:  Suppose the input is 6 bits wide, signed, with 2 fractional bits, and the output is forced to unsigned with 0 fractional bits.  Then an input of -2.0 (1110.00 in binary 2's complement) becomes an output of 56 (111000 in binary)."
  bus_out : Outport
  wires:
  concatenate/1 -> bus_out/1
  in1/1 -> reinterpret1/1
  reinterpret1/1 -> concatenate/1
  in2/1 -> reinterpret2/1
  reinterpret2/1 -> concatenate/2
  in3/1 -> reinterpret3/1
  reinterpret3/1 -> concatenate/3
  in4/1 -> reinterpret4/1
  reinterpret4/1 -> concatenate/4
  in5/1 -> reinterpret5/1
  reinterpret5/1 -> concatenate/5
  in6/1 -> reinterpret6/1
  reinterpret6/1 -> concatenate/6
  in7/1 -> reinterpret7/1
  reinterpret7/1 -> concatenate/7
  in8/1 -> reinterpret8/1
  reinterpret8/1 -> concatenate/8
  in9/1 -> reinterpret9/1
  reinterpret9/1 -> concatenate/9
  in10/1 -> reinterpret10/1
  reinterpret10/1 -> concatenate/10
  in11/1 -> reinterpret11/1
  reinterpret11/1 -> concatenate/11
  in12/1 -> reinterpret12/1
  reinterpret12/1 -> concatenate/12
  in13/1 -> reinterpret13/1
  reinterpret13/1 -> concatenate/13
  in14/1 -> reinterpret14/1
  reinterpret14/1 -> concatenate/14
  in15/1 -> reinterpret15/1
  reinterpret15/1 -> concatenate/15
  in16/1 -> reinterpret16/1
  reinterpret16/1 -> concatenate/16
  in17/1 -> reinterpret17/1
  reinterpret17/1 -> concatenate/17
  in18/1 -> reinterpret18/1
  reinterpret18/1 -> concatenate/18
  in19/1 -> reinterpret19/1
  reinterpret19/1 -> concatenate/19
  in20/1 -> reinterpret20/1
  reinterpret20/1 -> concatenate/20
  in21/1 -> reinterpret21/1
  reinterpret21/1 -> concatenate/21
  in22/1 -> reinterpret22/1
  reinterpret22/1 -> concatenate/22
  in23/1 -> reinterpret23/1
  reinterpret23/1 -> concatenate/23
  in24/1 -> reinterpret24/1
  reinterpret24/1 -> concatenate/24
  in25/1 -> reinterpret25/1
  reinterpret25/1 -> concatenate/25
  in26/1 -> reinterpret26/1
  reinterpret26/1 -> concatenate/26
  in27/1 -> reinterpret27/1
  reinterpret27/1 -> concatenate/27
  in28/1 -> reinterpret28/1
  reinterpret28/1 -> concatenate/28
  in29/1 -> reinterpret29/1
  reinterpret29/1 -> concatenate/29
  in30/1 -> reinterpret30/1
  reinterpret30/1 -> concatenate/30
  in31/1 -> reinterpret31/1
  reinterpret31/1 -> concatenate/31
  in32/1 -> reinterpret32/1
  reinterpret32/1 -> concatenate/32
  in33/1 -> reinterpret33/1
  reinterpret33/1 -> concatenate/33
  in34/1 -> reinterpret34/1
  reinterpret34/1 -> concatenate/34
  in35/1 -> reinterpret35/1
  reinterpret35/1 -> concatenate/35
  in36/1 -> reinterpret36/1
  reinterpret36/1 -> concatenate/36
  in37/1 -> reinterpret37/1
  reinterpret37/1 -> concatenate/37
  in38/1 -> reinterpret38/1
  reinterpret38/1 -> concatenate/38
  in39/1 -> reinterpret39/1
  reinterpret39/1 -> concatenate/39
  in40/1 -> reinterpret40/1
  reinterpret40/1 -> concatenate/40
  in41/1 -> reinterpret41/1
  reinterpret41/1 -> concatenate/41
  in42/1 -> reinterpret42/1
  reinterpret42/1 -> concatenate/42
  in43/1 -> reinterpret43/1
  reinterpret43/1 -> concatenate/43
  in44/1 -> reinterpret44/1
  reinterpret44/1 -> concatenate/44
  in45/1 -> reinterpret45/1
  reinterpret45/1 -> concatenate/45
  in46/1 -> reinterpret46/1
  reinterpret46/1 -> concatenate/46
  in47/1 -> reinterpret47/1
  reinterpret47/1 -> concatenate/47
  in48/1 -> reinterpret48/1
  reinterpret48/1 -> concatenate/48
  in49/1 -> reinterpret49/1
  reinterpret49/1 -> concatenate/49
  in50/1 -> reinterpret50/1
  reinterpret50/1 -> concatenate/50
  in51/1 -> reinterpret51/1
  reinterpret51/1 -> concatenate/51
  in52/1 -> reinterpret52/1
  reinterpret52/1 -> concatenate/52
  in53/1 -> reinterpret53/1
  reinterpret53/1 -> concatenate/53
  in54/1 -> reinterpret54/1
  reinterpret54/1 -> concatenate/54
  in55/1 -> reinterpret55/1
  reinterpret55/1 -> concatenate/55
  in56/1 -> reinterpret56/1
  reinterpret56/1 -> concatenate/56
  in57/1 -> reinterpret57/1
  reinterpret57/1 -> concatenate/57
  in58/1 -> reinterpret58/1
  reinterpret58/1 -> concatenate/58
  in59/1 -> reinterpret59/1
  reinterpret59/1 -> concatenate/59
  in60/1 -> reinterpret60/1
  reinterpret60/1 -> concatenate/60
  in61/1 -> reinterpret61/1
  reinterpret61/1 -> concatenate/61
  in62/1 -> reinterpret62/1
  reinterpret62/1 -> concatenate/62
  in63/1 -> reinterpret63/1
  reinterpret63/1 -> concatenate/63
  in64/1 -> reinterpret64/1
  reinterpret64/1 -> concatenate/64
